simulink model "Retry"  (R2019b)
settings: Solver=VariableStepAuto  StartTime=0.0  StopTime=10.0  RelTol=1e-3
settings Model: Creator=Sophia  LastModifiedBy=Sophia

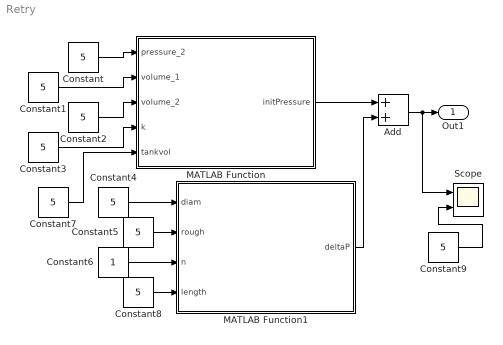
== system Retry ==
  Add : Sum
  Constant{,1..5,7..9} (9 alike) : Constant  Value=5
  Constant6 : Constant
  MATLAB Function : MATLAB Function  TreatAsAtomicUnit=on
  MATLAB Function1 : MATLAB Function  TreatAsAtomicUnit=on
  Scope : Scope  NumInputPorts=2
  Out1 : Outport
  wires:
  Constant/1 -> MATLAB Function/1(pressure_2)
  Constant3/1 -> MATLAB Function/4(k)
  Constant2/1 -> MATLAB Function/3(volume_2)
  Constant1/1 -> MATLAB Function/2(volume_1)
  MATLAB Function/1(initPressure) -> Add/1
  MATLAB Function1/1(deltaP) -> Add/2
  Constant4/1 -> MATLAB Function1/1(diam)
  Constant5/1 -> MATLAB Function1/2(rough)
  Constant6/1 -> MATLAB Function1/3(n)
  Add/1 -> Scope/1, Out1/1
  Constant8/1 -> MATLAB Function1/4(length)
  Constant9/1 -> Scope/2
  Constant7/1 -> MATLAB Function/5(tankvol)

== matlab function Retry/MATLAB Function1 ==
  data: diam input; rough input; deltaP output; n input; length input
%% Functions
function deltaP = getPressureDrop(diam, rough, n, length)
deltaP = zeros(1,100);
% Parameters
mdot = 0.9133; % kg/s
density = 786; % kg/m^3
dvisc = 0.00196; % dynamic viscosity, kg/m*s
kvisc = dvisc/density; % kinematic viscosity, m^2/s
len = length; % m
g = 9.81; % m/s^2
Q = mdot/density; % volumetric flow rate, m^3/s
diam = diam/39.37; % convert inches to meters
numPoints = n;
    for i=1:numPoints
        V = Q/(pi*(diam(i)/2)^2); % average velocity
        re = V*diam(i)/kvisc; % Reynolds number
        ed = rough/diam(i); % relative roughness
        ff = (1/(-1.8*log10((6.9/re)+(ed/3.7)^1.11)))^2; % friction factor
        hf = ff*len*(V^2)/(diam(i)*2*g); % head loss
        deltaP(i) = (density*g*hf)/(1e06); % pressure drop in MPa
        if i==1
           parameters = {'Diameter'; 'Average velocity (V)'; ...
               'Reynolds number (Re)'; 'Relative roughness (e/d)'; ...
               'Friction factor (f)'; 'Head loss (hf)'; ...
               'Pressure drop (delta P)'};
           Value = {diam(i); V; re; ed; ff; hf; deltaP(i)};
           Unit = {'m'; 'm/s'; 'None'; 'None'; 'None'; 'm'; 'Pa'};
%            example = table(Value, Unit, 'RowNames', parameters);
%            fprintf('Example calculation for i=%d: \n', i);
%            disp(example);
        end
    end
end

== matlab function Retry/MATLAB Function ==
  data: pressure_2 input; volume_1 input; initPressure output; volume_2 input; k input; tankvol input
function initPressure = fcn(pressure_2, volume_1, volume_2,k,tankvol)


%% God help Huzel & Huang R.I.P @95 years old
% Simple tank pressure requirement calculation assuming isentropic flow
% Jason Chen, 05 October, 2019

%% Simple Tank Pressure Calculation
% Using two isentropic expansion formulas
% https://www.grc.nasa.gov/www/k-12/airplane/compexp.html
numPoints = 100;
finalPressure = 1.6e06; % Final pressure inside tank
waterVolume = 4.567; % Liters
initVolume = linspace(waterVolume, 100-waterVolume, numPoints);
totalVolume = initVolume+waterVolume;
initTemp = 298; % Kevlin, room temperature
gamma = 1.40; % Ratio of specific heats of nitrogen gas
initPressures = zeros(1, numPoints);
finalTemps = zeros(1, numPoints);
for i=1:size(initVolume,2)
    v1 = initVolume(i);
    v2 = totalVolume(i);
    p2 = finalPressure;
    p1 = getInitPressure(p2, v1, v2, gamma);
    t1 = initTemp;
    t2 = getFinalTemp(t1, p1, p2, gamma);
    initPressures(i) = p1/1e06;
    finalTemps(i) = t2;
end    


%% Inputted Tank Volume
totalTankVolume = tankvol;
initPressurantVolume = totalTankVolume - 4.567;
finalPressure = 1.6e06;
initPressure = getInitPressure(finalPressure, initPressurantVolume, totalTankVolume, gamma);
finalTemp = getFinalTemp(initTemp, initPressurantVolume, totalTankVolume, gamma);
%disp("Initial Pressurant Pressure (MPa): " + initPressure/1e06);
%disp("Final Tank Temperature (K): " + finalTemp);
%% Functions
function finalTemp = getFinalTemp(temp_1, pressure_1, pressure_2, gamma)
    finalTemp = temp_1*(pressure_2/pressure_1)^((gamma-1)/gamma);
end
function initPressure = getInitPressure(pressure_2, volume_1, volume_2, k)
    initPressure = (pressure_2)/(volume_1/volume_2)^k;
end
end
